simulink subsystem "LogModule"  (R2024b)
settings: Solver=VariableStepAuto  StartTime=0.0  StopTime=10.0  RelTol=1e-3
undefined symbols (not defined in the file or in its folder): EgoState, FunctionOutput, RadarOutput, TargetState, TrackerOutput
settings Model: Creator=Tong  LastModifiedBy=Tong

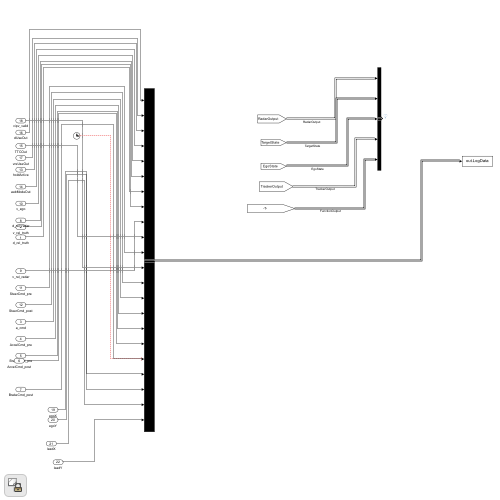
[thumbnail: Simulink's stored preview of the top-level diagram]
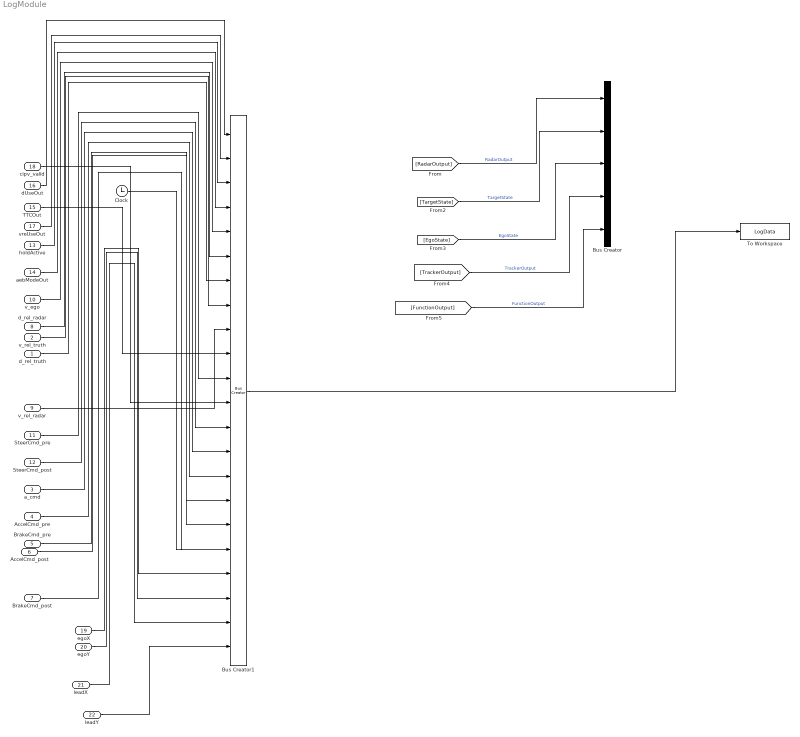
== system LogModule ==
  d_rel_truth : Inport
  v_rel_truth : Inport  Port=2
  a_cmd : Inport  Port=3
  AccelCmd_pre : Inport  Port=4
  BrakeCmd_pre : Inport  Port=5
  AccelCmd_post : Inport  Port=6
  BrakeCmd_post : Inport  Port=7
  d_rel_radar : Inport  Port=8
  v_rel_radar : Inport  Port=9
  v_ego : Inport  Port=10
  SteerCmd_pre : Inport  Port=11
  SteerCmd_post : Inport  Port=12
  holdActive : Inport  Port=13
  aebModeOut : Inport  Port=14
  TTCOut : Inport  Port=15
  dUseOut : Inport  Port=16
  vreUseOut : Inport  Port=17
  cipv_valid : Inport  Port=18
  egoX : Inport  Port=19
  egoY : Inport  Port=20
  leadX : Inport  Port=21
  leadY : Inport  Port=22
  Bus Creator : BusCreator  Inputs=RadarOutput,TargetState,EgoState,TrackerOutput,FunctionOutput
  Bus Creator1 : BusCreator  Inputs=22
  Clock : Clock
  To Workspace : ToWorkspace  VariableName=LogData  SaveFormat=Timeseries  SampleTime=-1
  wires:
  [RadarOutput] -> Bus Creator/1  "RadarOutput"
  [TargetState] -> Bus Creator/2  "TargetState"
  [EgoState] -> Bus Creator/3  "EgoState"
  [TrackerOutput] -> Bus Creator/4  "TrackerOutput"
  [FunctionOutput] -> Bus Creator/5  "FunctionOutput"
  Clock/1 -> ?
  cipv_valid/1 -> Bus Creator1/12
  dUseOut/1 -> Bus Creator1/1
  TTCOut/1 -> Bus Creator1/10
  vreUseOut/1 -> Bus Creator1/2
  holdActive/1 -> Bus Creator1/3
  aebModeOut/1 -> Bus Creator1/4
  v_ego/1 -> Bus Creator1/5
  d_rel_radar/1 -> Bus Creator1/6
  d_rel_truth/1 -> Bus Creator1/7
  v_rel_truth/1 -> Bus Creator1/8
  v_rel_radar/1 -> Bus Creator1/9
  SteerCmd_pre/1 -> Bus Creator1/11
  SteerCmd_post/1 -> Bus Creator1/13
  a_cmd/1 -> Bus Creator1/14
  AccelCmd_pre/1 -> Bus Creator1/15
  BrakeCmd_pre/1 -> Bus Creator1/16
  AccelCmd_post/1 -> Bus Creator1/17
  BrakeCmd_post/1 -> Bus Creator1/18
  Bus Creator1/1 -> To Workspace/1
  egoY/1 -> Bus Creator1/20
  egoX/1 -> Bus Creator1/19
  leadX/1 -> Bus Creator1/21
  leadY/1 -> Bus Creator1/22
